simulink library "sm_trackV_lib_belt_track_s45"  (R2026a)
settings: Solver=VariableStepAuto
undefined symbols (not defined in the file): carc_line_clr, carc_line_opc, L01, L02, L03, L04, L05, L06, L07, L08, L09, L1, L10, L11, L12, L13, L14, L15, L16, L17, L18, L19, L2, L20, L21, L22, L23, L24, L25, L26, L27, L28, L29, L3, L30, L31, L32, L33, L34, L35, L36, L37, L38, L39, L4, L40, L41, L42, L43, L44, L45, L5, L6, L7, L8, L9, lug_line_clr, lug_line_opc, T01, T02 ... (+45)
libraries: sm_trackV_lib_belt_segment x90
(part 2 of 2)

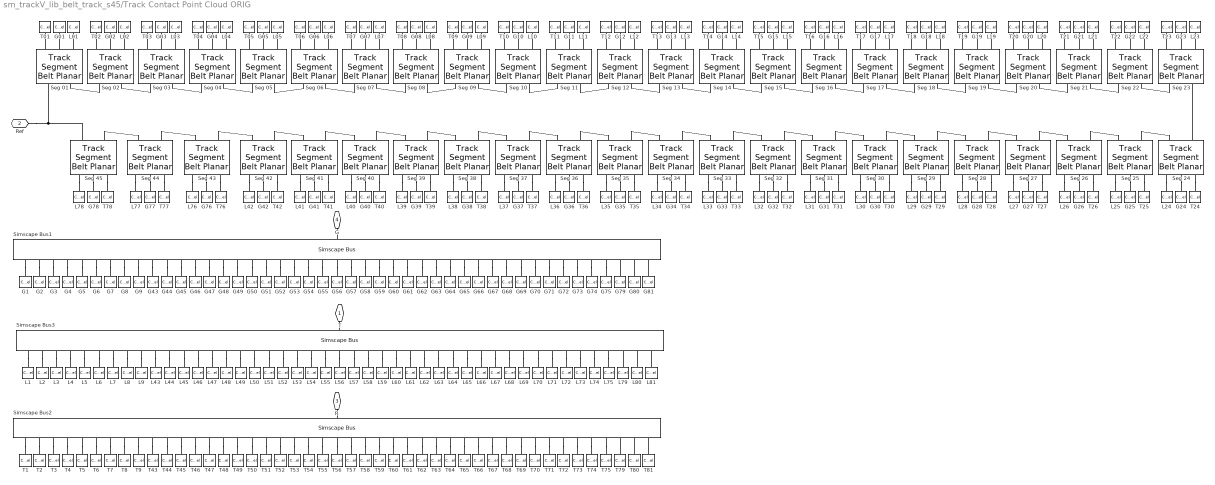
== system sm_trackV_lib_belt_track_s45/Track Contact Point Cloud ORIG ==
  G01 : ConnectionLabel  Label=G01
  G02 : ConnectionLabel  Label=G02
  G03 : ConnectionLabel  Label=G03
  G04 : ConnectionLabel  Label=G04
  G05 : ConnectionLabel  Label=G05
  G06 : ConnectionLabel  Label=G06
  G07 : ConnectionLabel  Label=G07
  G08 : ConnectionLabel  Label=G08
  G09 : ConnectionLabel  Label=G09
  G1 : ConnectionLabel  Label=G01
  G10 : ConnectionLabel  Label=G10
  G11 : ConnectionLabel  Label=G11
  G12 : ConnectionLabel  Label=G12
  G13 : ConnectionLabel  Label=G13
  G14 : ConnectionLabel  Label=G14
  G15 : ConnectionLabel  Label=G15
  G16 : ConnectionLabel  Label=G16
  G17 : ConnectionLabel  Label=G17
  G18 : ConnectionLabel  Label=G18
  G19 : ConnectionLabel  Label=G19
  G2 : ConnectionLabel  Label=G02
  G20 : ConnectionLabel  Label=G20
  G21 : ConnectionLabel  Label=G21
  G22 : ConnectionLabel  Label=G22
  G23 : ConnectionLabel  Label=G23
  G24 : ConnectionLabel  Label=G24
  G25 : ConnectionLabel  Label=G25
  G26 : ConnectionLabel  Label=G26
  G27 : ConnectionLabel  Label=G27
  G28 : ConnectionLabel  Label=G28
  G29 : ConnectionLabel  Label=G29
  G3 : ConnectionLabel  Label=G03
  G30 : ConnectionLabel  Label=G30
  G31 : ConnectionLabel  Label=G31
  G32 : ConnectionLabel  Label=G32
  G33 : ConnectionLabel  Label=G33
  G34 : ConnectionLabel  Label=G34
  G35 : ConnectionLabel  Label=G35
  G36 : ConnectionLabel  Label=G36
  G37 : ConnectionLabel  Label=G37
  G38 : ConnectionLabel  Label=G38
  G39 : ConnectionLabel  Label=G39
  G4 : ConnectionLabel  Label=G04
  G40 : ConnectionLabel  Label=G40
  G41 : ConnectionLabel  Label=G41
  G42 : ConnectionLabel  Label=G42
  G43 : ConnectionLabel  Label=G10
  G44 : ConnectionLabel  Label=G11
  G45 : ConnectionLabel  Label=G12
  G46 : ConnectionLabel  Label=G13
  G47 : ConnectionLabel  Label=G14
  G48 : ConnectionLabel  Label=G15
  G49 : ConnectionLabel  Label=G16
  G5 : ConnectionLabel  Label=G05
  G50 : ConnectionLabel  Label=G17
  G51 : ConnectionLabel  Label=G18
  G52 : ConnectionLabel  Label=G19
  G53 : ConnectionLabel  Label=G20
  G54 : ConnectionLabel  Label=G21
  G55 : ConnectionLabel  Label=G22
  G56 : ConnectionLabel  Label=G23
  G57 : ConnectionLabel  Label=G24
  G58 : ConnectionLabel  Label=G25
  G59 : ConnectionLabel  Label=G26
  G6 : ConnectionLabel  Label=G06
  G60 : ConnectionLabel  Label=G27
  G61 : ConnectionLabel  Label=G28
  G62 : ConnectionLabel  Label=G29
  G63 : ConnectionLabel  Label=G30
  G64 : ConnectionLabel  Label=G31
  G65 : ConnectionLabel  Label=G32
  G66 : ConnectionLabel  Label=G33
  G67 : ConnectionLabel  Label=G34
  G68 : ConnectionLabel  Label=G35
  G69 : ConnectionLabel  Label=G36
  G7 : ConnectionLabel  Label=G07
  G70 : ConnectionLabel  Label=G37
  G71 : ConnectionLabel  Label=G38
  G72 : ConnectionLabel  Label=G39
  G73 : ConnectionLabel  Label=G40
  G74 : ConnectionLabel  Label=G41
  G75 : ConnectionLabel  Label=G42
  G76 : ConnectionLabel  Label=G43
  G77 : ConnectionLabel  Label=G44
  G78 : ConnectionLabel  Label=G45
  G79 : ConnectionLabel  Label=G43
  G8 : ConnectionLabel  Label=G08
  G80 : ConnectionLabel  Label=G44
  G81 : ConnectionLabel  Label=G45
  G9 : ConnectionLabel  Label=G09
  L01 : ConnectionLabel  Label=L01
  L02 : ConnectionLabel  Label=L02
  L03 : ConnectionLabel  Label=L03
  L04 : ConnectionLabel  Label=L04
  L05 : ConnectionLabel  Label=L05
  L06 : ConnectionLabel  Label=L06
  L07 : ConnectionLabel  Label=L07
  L08 : ConnectionLabel  Label=L08
  L09 : ConnectionLabel  Label=L09
  L1 : ConnectionLabel  Label=L01
  L10 : ConnectionLabel  Label=L10
  L11 : ConnectionLabel  Label=L11
  L12 : ConnectionLabel  Label=L12
  L13 : ConnectionLabel  Label=L13
  L14 : ConnectionLabel  Label=L14
  L15 : ConnectionLabel  Label=L15
  L16 : ConnectionLabel  Label=L16
  L17 : ConnectionLabel  Label=L17
  L18 : ConnectionLabel  Label=L18
  L19 : ConnectionLabel  Label=L19
  L2 : ConnectionLabel  Label=L02
  L20 : ConnectionLabel  Label=L20
  L21 : ConnectionLabel  Label=L21
  L22 : ConnectionLabel  Label=L22
  L23 : ConnectionLabel  Label=L23
  L24 : ConnectionLabel  Label=L24
  L25 : ConnectionLabel  Label=L25
  L26 : ConnectionLabel  Label=L26
  L27 : ConnectionLabel  Label=L27
  L28 : ConnectionLabel  Label=L28
  L29 : ConnectionLabel  Label=L29
  L3 : ConnectionLabel  Label=L03
  L30 : ConnectionLabel  Label=L30
  L31 : ConnectionLabel  Label=L31
  L32 : ConnectionLabel  Label=L32
  L33 : ConnectionLabel  Label=L33
  L34 : ConnectionLabel  Label=L34
  L35 : ConnectionLabel  Label=L35
  L36 : ConnectionLabel  Label=L36
  L37 : ConnectionLabel  Label=L37
  L38 : ConnectionLabel  Label=L38
  L39 : ConnectionLabel  Label=L39
  L4 : ConnectionLabel  Label=L04
  L40 : ConnectionLabel  Label=L40
  L41 : ConnectionLabel  Label=L41
  L42 : ConnectionLabel  Label=L42
  L43 : ConnectionLabel  Label=L10
  L44 : ConnectionLabel  Label=L11
  L45 : ConnectionLabel  Label=L12
  L46 : ConnectionLabel  Label=L13
  L47 : ConnectionLabel  Label=L14
  L48 : ConnectionLabel  Label=L15
  L49 : ConnectionLabel  Label=L16
  L5 : ConnectionLabel  Label=L05
  L50 : ConnectionLabel  Label=L17
  L51 : ConnectionLabel  Label=L18
  L52 : ConnectionLabel  Label=L19
  L53 : ConnectionLabel  Label=L20
  L54 : ConnectionLabel  Label=L21
  L55 : ConnectionLabel  Label=L22
  L56 : ConnectionLabel  Label=L23
  L57 : ConnectionLabel  Label=L24
  L58 : ConnectionLabel  Label=L25
  L59 : ConnectionLabel  Label=L26
  L6 : ConnectionLabel  Label=L06
  L60 : ConnectionLabel  Label=L27
  L61 : ConnectionLabel  Label=L28
  L62 : ConnectionLabel  Label=L29
  L63 : ConnectionLabel  Label=L30
  L64 : ConnectionLabel  Label=L31
  L65 : ConnectionLabel  Label=L32
  L66 : ConnectionLabel  Label=L33
  L67 : ConnectionLabel  Label=L34
  L68 : ConnectionLabel  Label=L35
  L69 : ConnectionLabel  Label=L36
  L7 : ConnectionLabel  Label=L07
  L70 : ConnectionLabel  Label=L37
  L71 : ConnectionLabel  Label=L38
  L72 : ConnectionLabel  Label=L39
  L73 : ConnectionLabel  Label=L40
  L74 : ConnectionLabel  Label=L41
  L75 : ConnectionLabel  Label=L42
  L76 : ConnectionLabel  Label=L43
  L77 : ConnectionLabel  Label=L44
  L78 : ConnectionLabel  Label=L45
  L79 : ConnectionLabel  Label=L43
  L8 : ConnectionLabel  Label=L08
  L80 : ConnectionLabel  Label=L44
  L81 : ConnectionLabel  Label=L45
  L9 : ConnectionLabel  Label=L09
  Seg 01 : sm_trackV_lib_belt_segment/Track Segment Belt Planar  carc_len=carc_len  carc_wid=carc_wid  carc_thk=carc_thk  carc_mass=carc_mass  carc_cg=carc_cg  carc_moi=carc_moi  carc_poi=carc_poi  carc_clr=carc_clr  carc_opc=carc_opc  lug_hei=lug_hei  lug_lb=lug_lb  lug_lt=lug_lt  lug_w=lug_w  lug_xc=lug_xc  lug_clr=lug_clr  lug_opc=lug_opc  posTgtSpecify=on  posTgtPriority=High  PositionTargetValue=18.9945  DampingCoefficient=trackDamping  lug_line_clr=lug_line_clr  lug_line_opc=lug_line_opc  carc_line_clr=carc_line_clr  carc_line_opc=carc_line_opc  ptcld_belt=ptcld_belt  ptcld_belt_rad=ptcld_belt_rad  ptcld_belt_clr=ptcld_belt_clr  ptcld_belt_opc=ptcld_belt_opc
  Seg 02 : sm_trackV_lib_belt_segment/Track Segment Belt Planar  carc_len=carc_len  carc_wid=carc_wid  carc_thk=carc_thk  carc_mass=carc_mass  carc_cg=carc_cg  carc_moi=carc_moi  carc_poi=carc_poi  carc_clr=carc_clr  carc_opc=carc_opc  lug_hei=lug_hei  lug_lb=lug_lb  lug_lt=lug_lt  lug_w=lug_w  lug_xc=lug_xc  lug_clr=lug_clr  lug_opc=lug_opc  posTgtSpecify=on  posTgtPriority=High  PositionTargetValue=18.9945  DampingCoefficient=trackDamping  lug_line_clr=lug_line_clr  lug_line_opc=lug_line_opc  carc_line_clr=carc_line_clr  carc_line_opc=carc_line_opc  ptcld_belt=Trac.Belt.ground_contact.ptcld.pts  ptcld_belt_rad=Trac.Belt.ground_contact.ptcld.rad  ptcld_belt_clr=Trac.Belt.ground_contact.ptcld.clr  ptcld_belt_opc=Trac.Belt.ground_contact.ptcld.opc
  Seg 03 : sm_trackV_lib_belt_segment/Track Segment Belt Planar  carc_len=carc_len  carc_wid=carc_wid  carc_thk=carc_thk  carc_mass=carc_mass  carc_cg=carc_cg  carc_moi=carc_moi  carc_poi=carc_poi  carc_clr=carc_clr  carc_opc=carc_opc  lug_hei=lug_hei  lug_lb=lug_lb  lug_lt=lug_lt  lug_w=lug_w  lug_xc=lug_xc  lug_clr=lug_clr  lug_opc=lug_opc  posTgtSpecify=on  posTgtPriority=High  PositionTargetValue=18.9945  DampingCoefficient=trackDamping  lug_line_clr=lug_line_clr  lug_line_opc=lug_line_opc  carc_line_clr=carc_line_clr  carc_line_opc=carc_line_opc  ptcld_belt=Trac.Belt.ground_contact.ptcld.pts  ptcld_belt_rad=Trac.Belt.ground_contact.ptcld.rad  ptcld_belt_clr=Trac.Belt.ground_contact.ptcld.clr  ptcld_belt_opc=Trac.Belt.ground_contact.ptcld.opc
  Seg 04 : sm_trackV_lib_belt_segment/Track Segment Belt Planar  carc_len=carc_len  carc_wid=carc_wid  carc_thk=carc_thk  carc_mass=carc_mass  carc_cg=carc_cg  carc_moi=carc_moi  carc_poi=carc_poi  carc_clr=carc_clr  carc_opc=carc_opc  lug_hei=lug_hei  lug_lb=lug_lb  lug_lt=lug_lt  lug_w=lug_w  lug_xc=lug_xc  lug_clr=lug_clr  lug_opc=lug_opc  posTgtSpecify=on  posTgtPriority=High  PositionTargetValue=9.4972  DampingCoefficient=trackDamping  lug_line_clr=lug_line_clr  lug_line_opc=lug_line_opc  carc_line_clr=carc_line_clr  carc_line_opc=carc_line_opc  ptcld_belt=Trac.Belt.ground_contact.ptcld.pts  ptcld_belt_rad=Trac.Belt.ground_contact.ptcld.rad  ptcld_belt_clr=Trac.Belt.ground_contact.ptcld.clr  ptcld_belt_opc=Trac.Belt.ground_contact.ptcld.opc
  Seg 05 : sm_trackV_lib_belt_segment/Track Segment Belt Planar  carc_len=carc_len  carc_wid=carc_wid  carc_thk=carc_thk  carc_mass=carc_mass  carc_cg=carc_cg  carc_moi=carc_moi  carc_poi=carc_poi  carc_clr=carc_clr  carc_opc=carc_opc  lug_hei=lug_hei  lug_lb=lug_lb  lug_lt=lug_lt  lug_w=lug_w  lug_xc=lug_xc  lug_clr=lug_clr  lug_opc=lug_opc  posTgtSpecify=on  posTgtPriority=High  PositionTargetValue=0  DampingCoefficient=trackDamping  lug_line_clr=lug_line_clr  lug_line_opc=lug_line_opc  carc_line_clr=carc_line_clr  carc_line_opc=carc_line_opc  ptcld_belt=Trac.Belt.ground_contact.ptcld.pts  ptcld_belt_rad=Trac.Belt.ground_contact.ptcld.rad  ptcld_belt_clr=Trac.Belt.ground_contact.ptcld.clr  ptcld_belt_opc=Trac.Belt.ground_contact.ptcld.opc
  Seg 06 : sm_trackV_lib_belt_segment/Track Segment Belt Planar  carc_len=carc_len  carc_wid=carc_wid  carc_thk=carc_thk  carc_mass=carc_mass  carc_cg=carc_cg  carc_moi=carc_moi  carc_poi=carc_poi  carc_clr=carc_clr  carc_opc=carc_opc  lug_hei=lug_hei  lug_lb=lug_lb  lug_lt=lug_lt  lug_w=lug_w  lug_xc=lug_xc  lug_clr=lug_clr  lug_opc=lug_opc  posTgtSpecify=on  posTgtPriority=High  PositionTargetValue=0  DampingCoefficient=trackDamping  lug_line_clr=lug_line_clr  lug_line_opc=lug_line_opc  carc_line_clr=carc_line_clr  carc_line_opc=carc_line_opc  ptcld_belt=Trac.Belt.ground_contact.ptcld.pts  ptcld_belt_rad=Trac.Belt.ground_contact.ptcld.rad  ptcld_belt_clr=Trac.Belt.ground_contact.ptcld.clr  ptcld_belt_opc=Trac.Belt.ground_contact.ptcld.opc
  Seg 07 : sm_trackV_lib_belt_segment/Track Segment Belt Planar  carc_len=carc_len  carc_wid=carc_wid  carc_thk=carc_thk  carc_mass=carc_mass  carc_cg=carc_cg  carc_moi=carc_moi  carc_poi=carc_poi  carc_clr=carc_clr  carc_opc=carc_opc  lug_hei=lug_hei  lug_lb=lug_lb  lug_lt=lug_lt  lug_w=lug_w  lug_xc=lug_xc  lug_clr=lug_clr  lug_opc=lug_opc  posTgtSpecify=on  posTgtPriority=High  PositionTargetValue=0  DampingCoefficient=trackDamping  lug_line_clr=lug_line_clr  lug_line_opc=lug_line_opc  carc_line_clr=carc_line_clr  carc_line_opc=carc_line_opc  ptcld_belt=Trac.Belt.ground_contact.ptcld.pts  ptcld_belt_rad=Trac.Belt.ground_contact.ptcld.rad  ptcld_belt_clr=Trac.Belt.ground_contact.ptcld.clr  ptcld_belt_opc=Trac.Belt.ground_contact.ptcld.opc
  Seg 08 : sm_trackV_lib_belt_segment/Track Segment Belt Planar  carc_len=carc_len  carc_wid=carc_wid  carc_thk=carc_thk  carc_mass=carc_mass  carc_cg=carc_cg  carc_moi=carc_moi  carc_poi=carc_poi  carc_clr=carc_clr  carc_opc=carc_opc  lug_hei=lug_hei  lug_lb=lug_lb  lug_lt=lug_lt  lug_w=lug_w  lug_xc=lug_xc  lug_clr=lug_clr  lug_opc=lug_opc  posTgtSpecify=on  posTgtPriority=High  PositionTargetValue=0  DampingCoefficient=trackDamping  lug_line_clr=lug_line_clr  lug_line_opc=lug_line_opc  carc_line_clr=carc_line_clr  carc_line_opc=carc_line_opc  ptcld_belt=Trac.Belt.ground_contact.ptcld.pts  ptcld_belt_rad=Trac.Belt.ground_contact.ptcld.rad  ptcld_belt_clr=Trac.Belt.ground_contact.ptcld.clr  ptcld_belt_opc=Trac.Belt.ground_contact.ptcld.opc
  Seg 09 : sm_trackV_lib_belt_segment/Track Segment Belt Planar  carc_len=carc_len  carc_wid=carc_wid  carc_thk=carc_thk  carc_mass=carc_mass  carc_cg=carc_cg  carc_moi=carc_moi  carc_poi=carc_poi  carc_clr=carc_clr  carc_opc=carc_opc  lug_hei=lug_hei  lug_lb=lug_lb  lug_lt=lug_lt  lug_w=lug_w  lug_xc=lug_xc  lug_clr=lug_clr  lug_opc=lug_opc  posTgtSpecify=on  posTgtPriority=High  PositionTargetValue=22.7934  DampingCoefficient=trackDamping  lug_line_clr=lug_line_clr  lug_line_opc=lug_line_opc  carc_line_clr=carc_line_clr  carc_line_opc=carc_line_opc  ptcld_belt=Trac.Belt.ground_contact.ptcld.pts  ptcld_belt_rad=Trac.Belt.ground_contact.ptcld.rad  ptcld_belt_clr=Trac.Belt.ground_contact.ptcld.clr  ptcld_belt_opc=Trac.Belt.ground_contact.ptcld.opc
  Seg 10 : sm_trackV_lib_belt_segment/Track Segment Belt Planar  carc_len=carc_len  carc_wid=carc_wid  carc_thk=carc_thk  carc_mass=carc_mass  carc_cg=carc_cg  carc_moi=carc_moi  carc_poi=carc_poi  carc_clr=carc_clr  carc_opc=carc_opc  lug_hei=lug_hei  lug_lb=lug_lb  lug_lt=lug_lt  lug_w=lug_w  lug_xc=lug_xc  lug_clr=lug_clr  lug_opc=lug_opc  posTgtSpecify=on  posTgtPriority=High  PositionTargetValue=22.7934  DampingCoefficient=trackDamping  lug_line_clr=lug_line_clr  lug_line_opc=lug_line_opc  carc_line_clr=carc_line_clr  carc_line_opc=carc_line_opc  ptcld_belt=Trac.Belt.ground_contact.ptcld.pts  ptcld_belt_rad=Trac.Belt.ground_contact.ptcld.rad  ptcld_belt_clr=Trac.Belt.ground_contact.ptcld.clr  ptcld_belt_opc=Trac.Belt.ground_contact.ptcld.opc
  Seg 11 : sm_trackV_lib_belt_segment/Track Segment Belt Planar  carc_len=carc_len  carc_wid=carc_wid  carc_thk=carc_thk  carc_mass=carc_mass  carc_cg=carc_cg  carc_moi=carc_moi  carc_poi=carc_poi  carc_clr=carc_clr  carc_opc=carc_opc  lug_hei=lug_hei  lug_lb=lug_lb  lug_lt=lug_lt  lug_w=lug_w  lug_xc=lug_xc  lug_clr=lug_clr  lug_opc=lug_opc  posTgtSpecify=on  posTgtPriority=High  PositionTargetValue=22.7934  DampingCoefficient=trackDamping  lug_line_clr=lug_line_clr  lug_line_opc=lug_line_opc  carc_line_clr=carc_line_clr  carc_line_opc=carc_line_opc  ptcld_belt=Trac.Belt.ground_contact.ptcld.pts  ptcld_belt_rad=Trac.Belt.ground_contact.ptcld.rad  ptcld_belt_clr=Trac.Belt.ground_contact.ptcld.clr  ptcld_belt_opc=Trac.Belt.ground_contact.ptcld.opc
  Seg 12 : sm_trackV_lib_belt_segment/Track Segment Belt Planar  carc_len=carc_len  carc_wid=carc_wid  carc_thk=carc_thk  carc_mass=carc_mass  carc_cg=carc_cg  carc_moi=carc_moi  carc_poi=carc_poi  carc_clr=carc_clr  carc_opc=carc_opc  lug_hei=lug_hei  lug_lb=lug_lb  lug_lt=lug_lt  lug_w=lug_w  lug_xc=lug_xc  lug_clr=lug_clr  lug_opc=lug_opc  posTgtSpecify=on  posTgtPriority=High  PositionTargetValue=20.8939  DampingCoefficient=trackDamping  lug_line_clr=lug_line_clr  lug_line_opc=lug_line_opc  carc_line_clr=carc_line_clr  carc_line_opc=carc_line_opc  ptcld_belt=Trac.Belt.ground_contact.ptcld.pts  ptcld_belt_rad=Trac.Belt.ground_contact.ptcld.rad  ptcld_belt_clr=Trac.Belt.ground_contact.ptcld.clr  ptcld_belt_opc=Trac.Belt.ground_contact.ptcld.opc
  Seg 13 : sm_trackV_lib_belt_segment/Track Segment Belt Planar  carc_len=carc_len  carc_wid=carc_wid  carc_thk=carc_thk  carc_mass=carc_mass  carc_cg=carc_cg  carc_moi=carc_moi  carc_poi=carc_poi  carc_clr=carc_clr  carc_opc=carc_opc  lug_hei=lug_hei  lug_lb=lug_lb  lug_lt=lug_lt  lug_w=lug_w  lug_xc=lug_xc  lug_clr=lug_clr  lug_opc=lug_opc  posTgtSpecify=on  posTgtPriority=High  PositionTargetValue=14.2459  DampingCoefficient=trackDamping  lug_line_clr=lug_line_clr  lug_line_opc=lug_line_opc  carc_line_clr=carc_line_clr  carc_line_opc=carc_line_opc  ptcld_belt=Trac.Belt.ground_contact.ptcld.pts  ptcld_belt_rad=Trac.Belt.ground_contact.ptcld.rad  ptcld_belt_clr=Trac.Belt.ground_contact.ptcld.clr  ptcld_belt_opc=Trac.Belt.ground_contact.ptcld.opc
  Seg {14..26,33..44} (25 alike) : sm_trackV_lib_belt_segment/Track Segment Belt Planar  carc_len=carc_len  carc_wid=carc_wid  carc_thk=carc_thk  carc_mass=carc_mass  carc_cg=carc_cg  carc_moi=carc_moi  carc_poi=carc_poi  carc_clr=carc_clr  carc_opc=carc_opc  lug_hei=lug_hei  lug_lb=lug_lb  lug_lt=lug_lt  lug_w=lug_w  lug_xc=lug_xc  lug_clr=lug_clr  lug_opc=lug_opc  posTgtSpecify=on  posTgtPriority=High  PositionTargetValue=0  DampingCoefficient=trackDamping  lug_line_clr=lug_line_clr  lug_line_opc=lug_line_opc  carc_line_clr=carc_line_clr  carc_line_opc=carc_line_opc  ptcld_belt=Trac.Belt.ground_contact.ptcld.pts  ptcld_belt_rad=Trac.Belt.ground_contact.ptcld.rad  ptcld_belt_clr=Trac.Belt.ground_contact.ptcld.clr  ptcld_belt_opc=Trac.Belt.ground_contact.ptcld.opc
  Seg 27 : sm_trackV_lib_belt_segment/Track Segment Belt Planar  carc_len=carc_len  carc_wid=carc_wid  carc_thk=carc_thk  carc_mass=carc_mass  carc_cg=carc_cg  carc_moi=carc_moi  carc_poi=carc_poi  carc_clr=carc_clr  carc_opc=carc_opc  lug_hei=lug_hei  lug_lb=lug_lb  lug_lt=lug_lt  lug_w=lug_w  lug_xc=lug_xc  lug_clr=lug_clr  lug_opc=lug_opc  posTgtSpecify=on  posTgtPriority=Low  PositionTargetValue=0  DampingCoefficient=trackDamping  lug_line_clr=lug_line_clr  lug_line_opc=lug_line_opc  carc_line_clr=carc_line_clr  carc_line_opc=carc_line_opc  ptcld_belt=Trac.Belt.ground_contact.ptcld.pts  ptcld_belt_rad=Trac.Belt.ground_contact.ptcld.rad  ptcld_belt_clr=Trac.Belt.ground_contact.ptcld.clr  ptcld_belt_opc=Trac.Belt.ground_contact.ptcld.opc
  Seg 28 : sm_trackV_lib_belt_segment/Track Segment Belt Planar  carc_len=carc_len  carc_wid=carc_wid  carc_thk=carc_thk  carc_mass=carc_mass  carc_cg=carc_cg  carc_moi=carc_moi  carc_poi=carc_poi  carc_clr=carc_clr  carc_opc=carc_opc  lug_hei=lug_hei  lug_lb=lug_lb  lug_lt=lug_lt  lug_w=lug_w  lug_xc=lug_xc  lug_clr=lug_clr  lug_opc=lug_opc  posTgtSpecify=on  posTgtPriority=Low  PositionTargetValue=0  DampingCoefficient=trackDamping  lug_line_clr=lug_line_clr  lug_line_opc=lug_line_opc  carc_line_clr=carc_line_clr  carc_line_opc=carc_line_opc  ptcld_belt=Trac.Belt.ground_contact.ptcld.pts  ptcld_belt_rad=Trac.Belt.ground_contact.ptcld.rad  ptcld_belt_clr=Trac.Belt.ground_contact.ptcld.clr  ptcld_belt_opc=Trac.Belt.ground_contact.ptcld.opc
  Seg 29 : sm_trackV_lib_belt_segment/Track Segment Belt Planar  carc_len=carc_len  carc_wid=carc_wid  carc_thk=carc_thk  carc_mass=carc_mass  carc_cg=carc_cg  carc_moi=carc_moi  carc_poi=carc_poi  carc_clr=carc_clr  carc_opc=carc_opc  lug_hei=lug_hei  lug_lb=lug_lb  lug_lt=lug_lt  lug_w=lug_w  lug_xc=lug_xc  lug_clr=lug_clr  lug_opc=lug_opc  posTgtSpecify=on  posTgtPriority=Low  PositionTargetValue=0  DampingCoefficient=trackDamping  lug_line_clr=lug_line_clr  lug_line_opc=lug_line_opc  carc_line_clr=carc_line_clr  carc_line_opc=carc_line_opc  ptcld_belt=Trac.Belt.ground_contact.ptcld.pts  ptcld_belt_rad=Trac.Belt.ground_contact.ptcld.rad  ptcld_belt_clr=Trac.Belt.ground_contact.ptcld.clr  ptcld_belt_opc=Trac.Belt.ground_contact.ptcld.opc
  Seg 30 : sm_trackV_lib_belt_segment/Track Segment Belt Planar  carc_len=carc_len  carc_wid=carc_wid  carc_thk=carc_thk  carc_mass=carc_mass  carc_cg=carc_cg  carc_moi=carc_moi  carc_poi=carc_poi  carc_clr=carc_clr  carc_opc=carc_opc  lug_hei=lug_hei  lug_lb=lug_lb  lug_lt=lug_lt  lug_w=lug_w  lug_xc=lug_xc  lug_clr=lug_clr  lug_opc=lug_opc  posTgtSpecify=off  posTgtPriority=Low  PositionTargetValue=22.7934  DampingCoefficient=trackDamping  lug_line_clr=lug_line_clr  lug_line_opc=lug_line_opc  carc_line_clr=carc_line_clr  carc_line_opc=carc_line_opc  ptcld_belt=Trac.Belt.ground_contact.ptcld.pts  ptcld_belt_rad=Trac.Belt.ground_contact.ptcld.rad  ptcld_belt_clr=Trac.Belt.ground_contact.ptcld.clr  ptcld_belt_opc=Trac.Belt.ground_contact.ptcld.opc
  Seg 31 : sm_trackV_lib_belt_segment/Track Segment Belt Planar  carc_len=carc_len  carc_wid=carc_wid  carc_thk=carc_thk  carc_mass=carc_mass  carc_cg=carc_cg  carc_moi=carc_moi  carc_poi=carc_poi  carc_clr=carc_clr  carc_opc=carc_opc  lug_hei=lug_hei  lug_lb=lug_lb  lug_lt=lug_lt  lug_w=lug_w  lug_xc=lug_xc  lug_clr=lug_clr  lug_opc=lug_opc  posTgtSpecify=off  posTgtPriority=Low  PositionTargetValue=22.7934  DampingCoefficient=trackDamping  lug_line_clr=lug_line_clr  lug_line_opc=lug_line_opc  carc_line_clr=carc_line_clr  carc_line_opc=carc_line_opc  ptcld_belt=Trac.Belt.ground_contact.ptcld.pts  ptcld_belt_rad=Trac.Belt.ground_contact.ptcld.rad  ptcld_belt_clr=Trac.Belt.ground_contact.ptcld.clr  ptcld_belt_opc=Trac.Belt.ground_contact.ptcld.opc
  Seg 32 : sm_trackV_lib_belt_segment/Track Segment Belt Planar  carc_len=carc_len  carc_wid=carc_wid  carc_thk=carc_thk  carc_mass=carc_mass  carc_cg=carc_cg  carc_moi=carc_moi  carc_poi=carc_poi  carc_clr=carc_clr  carc_opc=carc_opc  lug_hei=lug_hei  lug_lb=lug_lb  lug_lt=lug_lt  lug_w=lug_w  lug_xc=lug_xc  lug_clr=lug_clr  lug_opc=lug_opc  posTgtSpecify=off  posTgtPriority=Low  PositionTargetValue=22.7934  DampingCoefficient=trackDamping  lug_line_clr=lug_line_clr  lug_line_opc=lug_line_opc  carc_line_clr=carc_line_clr  carc_line_opc=carc_line_opc  ptcld_belt=Trac.Belt.ground_contact.ptcld.pts  ptcld_belt_rad=Trac.Belt.ground_contact.ptcld.rad  ptcld_belt_clr=Trac.Belt.ground_contact.ptcld.clr  ptcld_belt_opc=Trac.Belt.ground_contact.ptcld.opc
  Seg 45 : sm_trackV_lib_belt_segment/Track Segment Belt Planar  carc_len=carc_len  carc_wid=carc_wid  carc_thk=carc_thk  carc_mass=carc_mass  carc_cg=carc_cg  carc_moi=carc_moi  carc_poi=carc_poi  carc_clr=carc_clr  carc_opc=carc_opc  lug_hei=lug_hei  lug_lb=lug_lb  lug_lt=lug_lt  lug_w=lug_w  lug_xc=lug_xc  lug_clr=lug_clr  lug_opc=lug_opc  posTgtSpecify=on  posTgtPriority=High  PositionTargetValue=9.4972  DampingCoefficient=trackDamping  lug_line_clr=lug_line_clr  lug_line_opc=lug_line_opc  carc_line_clr=carc_line_clr  carc_line_opc=carc_line_opc  ptcld_belt=Trac.Belt.ground_contact.ptcld.pts  ptcld_belt_rad=Trac.Belt.ground_contact.ptcld.rad  ptcld_belt_clr=Trac.Belt.ground_contact.ptcld.clr  ptcld_belt_opc=Trac.Belt.ground_contact.ptcld.opc
  Simscape Bus1 : SimscapeBus  HierarchyStrings=T01;T02;T03;T04;T05;T06;T07;T08;T09;T10;T11;T12;T13;T14;T15;T16;T17;T18;T19;T20;T21;T22;T23;T24;T25;T26;T27;T28;T29;T30;T31;T32;T33;T34;T35;T36;T37;T38;T39;T40;T41;T42;T43;T44;T45  ConnectionType=Bus: CBO_TrRoll
  Simscape Bus2 : SimscapeBus  HierarchyStrings=T01;T02;T03;T04;T05;T06;T07;T08;T09;T10;T11;T12;T13;T14;T15;T16;T17;T18;T19;T20;T21;T22;T23;T24;T25;T26;T27;T28;T29;T30;T31;T32;T33;T34;T35;T36;T37;T38;T39;T40;T41;T42;T43;T44;T45  ConnectionType=Bus: CBO_TrRoll
  Simscape Bus3 : SimscapeBus  HierarchyStrings=L01;L02;L03;L04;L05;L06;L07;L08;L09;L10;L11;L12;L13;L14;L15;L16;L17;L18;L19;L20;L21;L22;L23;L24;L25;L26;L27;L28;L29;L30;L31;L32;L33;L34;L35;L36;L37;L38;L39;L40;L41;L42;L43;L44;L45  ConnectionType=Bus: CBO_TrSpr
  T01 : ConnectionLabel  Label=T01
  T02 : ConnectionLabel  Label=T02
  T03 : ConnectionLabel  Label=T03
  T04 : ConnectionLabel  Label=T04
  T05 : ConnectionLabel  Label=T05
  T06 : ConnectionLabel  Label=T06
  T07 : ConnectionLabel  Label=T07
  T08 : ConnectionLabel  Label=T08
  T09 : ConnectionLabel  Label=T09
  T1 : ConnectionLabel  Label=T01
  T10 : ConnectionLabel  Label=T10
  T11 : ConnectionLabel  Label=T11
  T12 : ConnectionLabel  Label=T12
  T13 : ConnectionLabel  Label=T13
  T14 : ConnectionLabel  Label=T14
  T15 : ConnectionLabel  Label=T15
  T16 : ConnectionLabel  Label=T16
  T17 : ConnectionLabel  Label=T17
  T18 : ConnectionLabel  Label=T18
  T19 : ConnectionLabel  Label=T19
  T2 : ConnectionLabel  Label=T02
  T20 : ConnectionLabel  Label=T20
  T21 : ConnectionLabel  Label=T21
  T22 : ConnectionLabel  Label=T22
  T23 : ConnectionLabel  Label=T23
  T24 : ConnectionLabel  Label=T24
  T25 : ConnectionLabel  Label=T25
  T26 : ConnectionLabel  Label=T26
  T27 : ConnectionLabel  Label=T27
  T28 : ConnectionLabel  Label=T28
  T29 : ConnectionLabel  Label=T29
  T3 : ConnectionLabel  Label=T03
  T30 : ConnectionLabel  Label=T30
  T31 : ConnectionLabel  Label=T31
  T32 : ConnectionLabel  Label=T32
  T33 : ConnectionLabel  Label=T33
  T34 : ConnectionLabel  Label=T34
  T35 : ConnectionLabel  Label=T35
  T36 : ConnectionLabel  Label=T36
  T37 : ConnectionLabel  Label=T37
  T38 : ConnectionLabel  Label=T38
  T39 : ConnectionLabel  Label=T39
  T4 : ConnectionLabel  Label=T04
  T40 : ConnectionLabel  Label=T40
  T41 : ConnectionLabel  Label=T41
  T42 : ConnectionLabel  Label=T42
  T43 : ConnectionLabel  Label=T10
  T44 : ConnectionLabel  Label=T11
  T45 : ConnectionLabel  Label=T12
  T46 : ConnectionLabel  Label=T13
  T47 : ConnectionLabel  Label=T14
  T48 : ConnectionLabel  Label=T15
  T49 : ConnectionLabel  Label=T16
  T5 : ConnectionLabel  Label=T05
  T50 : ConnectionLabel  Label=T17
  T51 : ConnectionLabel  Label=T18
  T52 : ConnectionLabel  Label=T19
  T53 : ConnectionLabel  Label=T20
  T54 : ConnectionLabel  Label=T21
  T55 : ConnectionLabel  Label=T22
  T56 : ConnectionLabel  Label=T23
  T57 : ConnectionLabel  Label=T24
  T58 : ConnectionLabel  Label=T25
  T59 : ConnectionLabel  Label=T26
  T6 : ConnectionLabel  Label=T06
  T60 : ConnectionLabel  Label=T27
  T61 : ConnectionLabel  Label=T28
  T62 : ConnectionLabel  Label=T29
  T63 : ConnectionLabel  Label=T30
  T64 : ConnectionLabel  Label=T31
  T65 : ConnectionLabel  Label=T32
  T66 : ConnectionLabel  Label=T33
  T67 : ConnectionLabel  Label=T34
  T68 : ConnectionLabel  Label=T35
  T69 : ConnectionLabel  Label=T36
  T7 : ConnectionLabel  Label=T07
  T70 : ConnectionLabel  Label=T37
  T71 : ConnectionLabel  Label=T38
  T72 : ConnectionLabel  Label=T39
  T73 : ConnectionLabel  Label=T40
  T74 : ConnectionLabel  Label=T41
  T75 : ConnectionLabel  Label=T42
  T76 : ConnectionLabel  Label=T43
  T77 : ConnectionLabel  Label=T44
  T78 : ConnectionLabel  Label=T45
  T79 : ConnectionLabel  Label=T43
  T8 : ConnectionLabel  Label=T08
  T80 : ConnectionLabel  Label=T44
  T81 : ConnectionLabel  Label=T45
  T9 : ConnectionLabel  Label=T09
  T : PMIOPort  Side=Right
  Ref : PMIOPort  Port=2  Side=Right
  R : PMIOPort  Port=3  Side=Right
  G : PMIOPort  Port=4  Side=Left
  connections:
  Ref/RConn1 -- Seg 45/LConn2 -- Seg 01/LConn1
  Seg 02/RConn3 -- L02/LConn1
  Seg 45/RConn2 -- G78/LConn1
  Simscape Bus1/LConn16 -- G49/LConn1
  Seg 19/LConn1 -- Seg 18/LConn2
  Simscape Bus2/LConn2 -- T2/LConn1
  Simscape Bus1/LConn1 -- G1/LConn1
  Simscape Bus2/LConn3 -- T3/LConn1
  Seg 34/LConn1 -- Seg 33/LConn2
  Simscape Bus3/LConn40 -- L73/LConn1
  Simscape Bus2/RConn1 -- R/RConn1
  Seg 01/RConn2 -- G01/LConn1
  Seg 05/RConn2 -- G05/LConn1
  Simscape Bus2/LConn40 -- T73/LConn1
  Seg 42/LConn1 -- Seg 41/LConn2
  Seg 24/RConn2 -- G24/LConn1
  Simscape Bus1/LConn27 -- G60/LConn1
  Simscape Bus1/LConn40 -- G73/LConn1
  Simscape Bus1/LConn39 -- G72/LConn1
  Seg 22/RConn3 -- L22/LConn1
  Seg 22/RConn2 -- G22/LConn1
  Seg 32/RConn3 -- L32/LConn1
  Simscape Bus1/LConn41 -- G74/LConn1
  Simscape Bus1/LConn33 -- G66/LConn1
  Simscape Bus1/LConn11 -- G44/LConn1
  Seg 22/RConn1 -- T22/LConn1
  Seg 06/RConn1 -- T06/LConn1
  Simscape Bus1/LConn22 -- G55/LConn1
  Simscape Bus1/LConn17 -- G50/LConn1
  Simscape Bus1/LConn20 -- G53/LConn1
  Simscape Bus2/LConn41 -- T74/LConn1
  Simscape Bus1/LConn23 -- G56/LConn1
  Seg 08/RConn2 -- G08/LConn1
  Seg 44/LConn1 -- Seg 43/LConn2
  Seg 15/LConn1 -- Seg 14/LConn2
  Simscape Bus1/LConn7 -- G7/LConn1
  Seg 13/RConn2 -- G13/LConn1
  Seg 05/RConn1 -- T05/LConn1
  Seg 25/RConn2 -- G25/LConn1
  Seg 28/LConn1 -- Seg 27/LConn2
  Seg 03/LConn1 -- Seg 02/LConn2
  Simscape Bus1/LConn15 -- G48/LConn1
  Seg 13/RConn3 -- L13/LConn1
  Seg 14/RConn1 -- T14/LConn1
  Seg 18/RConn2 -- G18/LConn1
  Simscape Bus1/LConn3 -- G3/LConn1
  Seg 08/LConn1 -- Seg 07/LConn2
  Seg 11/RConn2 -- G11/LConn1
  Seg 02/RConn1 -- T02/LConn1
  Simscape Bus2/LConn39 -- T72/LConn1
  Seg 21/LConn1 -- Seg 20/LConn2
  Seg 21/RConn1 -- T21/LConn1
  Seg 18/LConn1 -- Seg 17/LConn2
  Seg 08/RConn3 -- L08/LConn1
  Seg 34/RConn2 -- G34/LConn1
  Seg 30/LConn1 -- Seg 29/LConn2
  Seg 28/RConn1 -- T28/LConn1
  Seg 36/RConn3 -- L36/LConn1
  Seg 10/LConn2 -- Seg 11/LConn1
  Seg 01/RConn1 -- T01/LConn1
  Seg 33/LConn1 -- Seg 32/LConn2
  Seg 20/RConn1 -- T20/LConn1
  Seg 42/RConn3 -- L42/LConn1
  Simscape Bus2/LConn6 -- T6/LConn1
  Seg 16/RConn3 -- L16/LConn1
  Seg 27/RConn1 -- T27/LConn1
  Seg 04/LConn1 -- Seg 03/LConn2
  Simscape Bus1/LConn5 -- G5/LConn1
  Seg 39/RConn2 -- G39/LConn1
  Seg 09/RConn2 -- G09/LConn1
  Seg 07/RConn3 -- L07/LConn1
  Seg 26/RConn2 -- G26/LConn1
  Seg 41/RConn2 -- G41/LConn1
  Seg 26/LConn1 -- Seg 25/LConn2
  Seg 41/RConn3 -- L41/LConn1
  Seg 03/RConn1 -- T03/LConn1
  Seg 23/LConn1 -- Seg 22/LConn2
  Seg 31/RConn1 -- T31/LConn1
  Simscape Bus1/LConn4 -- G4/LConn1
  Seg 01/RConn3 -- L01/LConn1
  Simscape Bus1/RConn1 -- G/RConn1
  Seg 17/RConn2 -- G17/LConn1
  Seg 26/RConn3 -- L26/LConn1
  Seg 37/RConn1 -- T37/LConn1
  Simscape Bus3/LConn39 -- L72/LConn1
  Seg 43/LConn1 -- Seg 42/LConn2
  Simscape Bus2/LConn42 -- T75/LConn1
  Seg 43/RConn2 -- G76/LConn1
  Seg 30/RConn3 -- L30/LConn1
  Seg 43/RConn3 -- L76/LConn1
  Seg 33/RConn3 -- L33/LConn1
  Simscape Bus3/LConn27 -- L60/LConn1
  Simscape Bus3/LConn38 -- L71/LConn1
  Seg 31/RConn2 -- G31/LConn1
  Simscape Bus3/LConn31 -- L64/LConn1
  Seg 10/RConn2 -- G10/LConn1
  Seg 06/RConn2 -- G06/LConn1
  Simscape Bus1/LConn37 -- G70/LConn1
  Seg 17/LConn1 -- Seg 16/LConn2
  Seg 42/RConn2 -- G42/LConn1
  Simscape Bus3/LConn25 -- L58/LConn1
  Seg 34/RConn1 -- T34/LConn1
  Simscape Bus1/LConn30 -- G63/LConn1
  Seg 21/RConn3 -- L21/LConn1
  Simscape Bus3/LConn28 -- L61/LConn1
  Seg 24/LConn1 -- Seg 23/LConn2
  Seg 15/RConn1 -- T15/LConn1
  Seg 10/LConn1 -- Seg 09/LConn2
  Simscape Bus3/LConn20 -- L53/LConn1
  Seg 18/RConn1 -- T18/LConn1
  Seg 11/LConn2 -- Seg 12/LConn1
  Seg 40/RConn1 -- T40/LConn1
  Simscape Bus3/LConn30 -- L63/LConn1
  Seg 32/LConn1 -- Seg 31/LConn2
  Simscape Bus1/LConn19 -- G52/LConn1
  Simscape Bus3/LConn7 -- L7/LConn1
  Simscape Bus3/LConn8 -- L8/LConn1
  Simscape Bus3/LConn19 -- L52/LConn1
  Simscape Bus1/LConn10 -- G43/LConn1
  Simscape Bus3/LConn5 -- L5/LConn1
  Simscape Bus1/LConn28 -- G61/LConn1
  Seg 34/RConn3 -- L34/LConn1
  Seg 12/RConn2 -- G12/LConn1
  Seg 19/RConn3 -- L19/LConn1
  Simscape Bus3/LConn17 -- L50/LConn1
  Seg 24/RConn1 -- T24/LConn1
  Seg 07/RConn2 -- G07/LConn1
  Seg 42/RConn1 -- T42/LConn1
  Seg 41/RConn1 -- T41/LConn1
  Seg 37/LConn1 -- Seg 36/LConn2
  Seg 27/RConn3 -- L27/LConn1
  Seg 28/RConn2 -- G28/LConn1
  Seg 27/LConn1 -- Seg 26/LConn2
  Seg 13/RConn1 -- T13/LConn1
  Seg 45/LConn1 -- Seg 44/LConn2
  Seg 12/RConn1 -- T12/LConn1
  Seg 41/LConn1 -- Seg 40/LConn2
  Simscape Bus3/LConn18 -- L51/LConn1
  Simscape Bus1/LConn6 -- G6/LConn1
  Seg 20/RConn2 -- G20/LConn1
  Simscape Bus2/LConn9 -- T9/LConn1
  Seg 07/RConn1 -- T07/LConn1
  Simscape Bus2/LConn7 -- T7/LConn1
  Seg 28/RConn3 -- L28/LConn1
  Simscape Bus3/LConn23 -- L56/LConn1
  Seg 11/RConn1 -- T11/LConn1
  Simscape Bus1/LConn14 -- G47/LConn1
  Seg 03/RConn3 -- L03/LConn1
  Simscape Bus3/LConn15 -- L48/LConn1
  Seg 44/RConn3 -- L77/LConn1
  Simscape Bus3/LConn14 -- L47/LConn1
  Seg 35/RConn3 -- L35/LConn1
  Seg 04/RConn1 -- T04/LConn1
  Seg 23/RConn3 -- L23/LConn1
  Seg 38/RConn1 -- T38/LConn1
  Simscape Bus2/LConn5 -- T5/LConn1
  Simscape Bus2/LConn1 -- T1/LConn1
  Seg 24/RConn3 -- L24/LConn1
  Seg 32/RConn2 -- G32/LConn1
  Seg 03/RConn2 -- G03/LConn1
  Simscape Bus3/LConn37 -- L70/LConn1
  Simscape Bus1/LConn32 -- G65/LConn1
  Simscape Bus1/LConn36 -- G69/LConn1
  Simscape Bus1/LConn29 -- G62/LConn1
  Seg 37/RConn3 -- L37/LConn1
  Simscape Bus1/LConn34 -- G67/LConn1
  Simscape Bus3/LConn35 -- L68/LConn1
  Simscape Bus2/LConn28 -- T61/LConn1
  Seg 05/RConn3 -- L05/LConn1
  Seg 22/LConn1 -- Seg 21/LConn2
  Simscape Bus2/LConn8 -- T8/LConn1
  Seg 10/RConn1 -- T10/LConn1
  Seg 29/RConn3 -- L29/LConn1
  Seg 40/RConn2 -- G40/LConn1
  Simscape Bus2/LConn21 -- T54/LConn1
  Simscape Bus2/LConn22 -- T55/LConn1
  Seg 30/RConn2 -- G30/LConn1
  Simscape Bus3/LConn22 -- L55/LConn1
  Simscape Bus3/LConn9 -- L9/LConn1
  Seg 27/RConn2 -- G27/LConn1
  Seg 20/LConn1 -- Seg 19/LConn2
  Seg 05/LConn1 -- Seg 04/LConn2
  Seg 11/RConn3 -- L11/LConn1
  Simscape Bus3/RConn1 -- T/RConn1
  Seg 16/LConn1 -- Seg 15/LConn2
  Simscape Bus3/LConn4 -- L4/LConn1
  Seg 26/RConn1 -- T26/LConn1
  Seg 38/LConn1 -- Seg 37/LConn2
  Simscape Bus2/LConn17 -- T50/LConn1
  Seg 14/LConn1 -- Seg 13/LConn2
  Seg 09/RConn1 -- T09/LConn1
  Simscape Bus2/LConn19 -- T52/LConn1
  Seg 33/RConn2 -- G33/LConn1
  Simscape Bus1/LConn13 -- G46/LConn1
  Simscape Bus1/LConn2 -- G2/LConn1
  Simscape Bus3/LConn34 -- L67/LConn1
  Seg 09/RConn3 -- L09/LConn1
  Simscape Bus1/LConn25 -- G58/LConn1
  Simscape Bus2/LConn14 -- T47/LConn1
  Seg 14/RConn3 -- L14/LConn1
  Simscape Bus1/LConn38 -- G71/LConn1
  Simscape Bus3/LConn11 -- L44/LConn1
  Seg 39/LConn1 -- Seg 38/LConn2
  Seg 16/RConn1 -- T16/LConn1
  Simscape Bus2/LConn25 -- T58/LConn1
  Simscape Bus2/LConn12 -- T45/LConn1
  Seg 21/RConn2 -- G21/LConn1
  Simscape Bus3/LConn13 -- L46/LConn1
  Seg 15/RConn3 -- L15/LConn1
  Seg 29/LConn1 -- Seg 28/LConn2
  Simscape Bus1/LConn9 -- G9/LConn1
  Simscape Bus3/LConn12 -- L45/LConn1
  Seg 15/RConn2 -- G15/LConn1
  Seg 02/RConn2 -- G02/LConn1
  Simscape Bus2/LConn4 -- T4/LConn1
  Seg 07/LConn1 -- Seg 06/LConn2
  Seg 12/RConn3 -- L12/LConn1
  Seg 40/LConn1 -- Seg 39/LConn2
  Seg 39/RConn1 -- T39/LConn1
  Simscape Bus3/LConn24 -- L57/LConn1
  Simscape Bus2/LConn29 -- T62/LConn1
  Simscape Bus3/LConn33 -- L66/LConn1
  Seg 43/RConn1 -- T76/LConn1
  Seg 25/RConn1 -- T25/LConn1
  Simscape Bus3/LConn21 -- L54/LConn1
  Simscape Bus3/LConn2 -- L2/LConn1
  Simscape Bus1/LConn42 -- G75/LConn1
  Seg 16/RConn2 -- G16/LConn1
  Simscape Bus3/LConn1 -- L1/LConn1
  Seg 29/RConn1 -- T29/LConn1
  Seg 19/RConn2 -- G19/LConn1
  Simscape Bus1/LConn31 -- G64/LConn1
  Seg 31/RConn3 -- L31/LConn1
  Simscape Bus3/LConn29 -- L62/LConn1
  Simscape Bus1/LConn24 -- G57/LConn1
  Seg 33/RConn1 -- T33/LConn1
  Seg 32/RConn1 -- T32/LConn1
  Simscape Bus2/LConn23 -- T56/LConn1
  Simscape Bus1/LConn35 -- G68/LConn1
  Seg 37/RConn2 -- G37/LConn1
  Simscape Bus2/LConn18 -- T51/LConn1
  Simscape Bus2/LConn37 -- T70/LConn1
  Simscape Bus2/LConn33 -- T66/LConn1
  Simscape Bus2/LConn30 -- T63/LConn1
  Seg 38/RConn3 -- L38/LConn1
  Seg 25/RConn3 -- L25/LConn1
  Seg 29/RConn2 -- G29/LConn1
  Simscape Bus1/LConn18 -- G51/LConn1
  Simscape Bus3/LConn6 -- L6/LConn1
  Simscape Bus3/LConn26 -- L59/LConn1
  Simscape Bus2/LConn16 -- T49/LConn1
  Simscape Bus3/LConn16 -- L49/LConn1
  Simscape Bus2/LConn35 -- T68/LConn1
  Seg 17/RConn3 -- L17/LConn1
  Simscape Bus2/LConn36 -- T69/LConn1
  Simscape Bus2/LConn20 -- T53/LConn1
  Seg 36/RConn1 -- T36/LConn1
  Simscape Bus3/LConn3 -- L3/LConn1
  Seg 10/RConn3 -- L10/LConn1
  Seg 08/LConn2 -- Seg 09/LConn1
  Seg 06/RConn3 -- L06/LConn1
  Seg 40/RConn3 -- L40/LConn1
  Seg 05/LConn2 -- Seg 06/LConn1
  Seg 36/RConn2 -- G36/LConn1
  Simscape Bus3/LConn32 -- L65/LConn1
  Simscape Bus2/LConn10 -- T43/LConn1
  Seg 04/RConn2 -- G04/LConn1
  Simscape Bus2/LConn24 -- T57/LConn1
  Seg 23/RConn2 -- G23/LConn1
  Simscape Bus2/LConn32 -- T65/LConn1
  Simscape Bus2/LConn26 -- T59/LConn1
  Simscape Bus2/LConn31 -- T64/LConn1
  Seg 45/RConn3 -- L78/LConn1
  Simscape Bus1/LConn21 -- G54/LConn1
  Seg 08/RConn1 -- T08/LConn1
  Simscape Bus1/LConn26 -- G59/LConn1
  Seg 31/LConn1 -- Seg 30/LConn2
  Seg 35/RConn1 -- T35/LConn1
  Simscape Bus2/LConn38 -- T71/LConn1
  Simscape Bus2/LConn34 -- T67/LConn1
  Simscape Bus2/LConn27 -- T60/LConn1
  Seg 35/LConn1 -- Seg 34/LConn2
  Simscape Bus3/LConn10 -- L43/LConn1
  Simscape Bus2/LConn11 -- T44/LConn1
  Seg 19/RConn1 -- T19/LConn1
  Simscape Bus3/LConn36 -- L69/LConn1
  Seg 20/RConn3 -- L20/LConn1
  Seg 18/RConn3 -- L18/LConn1
  Seg 44/RConn2 -- G77/LConn1
  Seg 35/RConn2 -- G35/LConn1
  Seg 17/RConn1 -- T17/LConn1
  Simscape Bus1/LConn12 -- G45/LConn1
  Seg 30/RConn1 -- T30/LConn1
  Seg 39/RConn3 -- L39/LConn1
  Simscape Bus3/LConn42 -- L75/LConn1
  Seg 44/RConn1 -- T77/LConn1
  Seg 36/LConn1 -- Seg 35/LConn2
  Simscape Bus2/LConn13 -- T46/LConn1
  Seg 04/RConn3 -- L04/LConn1
  Seg 45/RConn1 -- T78/LConn1
  Simscape Bus2/LConn15 -- T48/LConn1
  Seg 38/RConn2 -- G38/LConn1
  Seg 13/LConn1 -- Seg 12/LConn2
  Simscape Bus1/LConn8 -- G8/LConn1
  Seg 23/RConn1 -- T23/LConn1
  Simscape Bus3/LConn41 -- L74/LConn1
  Seg 14/RConn2 -- G14/LConn1
  Seg 02/LConn1 -- Seg 01/LConn2
  Seg 25/LConn1 -- Seg 24/LConn2
  G79/LConn1 -- Simscape Bus1/LConn43
  G80/LConn1 -- Simscape Bus1/LConn44
  G81/LConn1 -- Simscape Bus1/LConn45
  L79/LConn1 -- Simscape Bus3/LConn43
  L80/LConn1 -- Simscape Bus3/LConn44
  L81/LConn1 -- Simscape Bus3/LConn45
  T79/LConn1 -- Simscape Bus2/LConn43
  T80/LConn1 -- Simscape Bus2/LConn44
  T81/LConn1 -- Simscape Bus2/LConn45
